simulink model "assignment_9"  (R2020b)
settings: Solver=VariableStepAuto  StartTime=0.0  StopTime=0.2  RelTol=1e-3
settings Model: Creator=Sudhanshu  LastModifiedBy=Sudhanshu

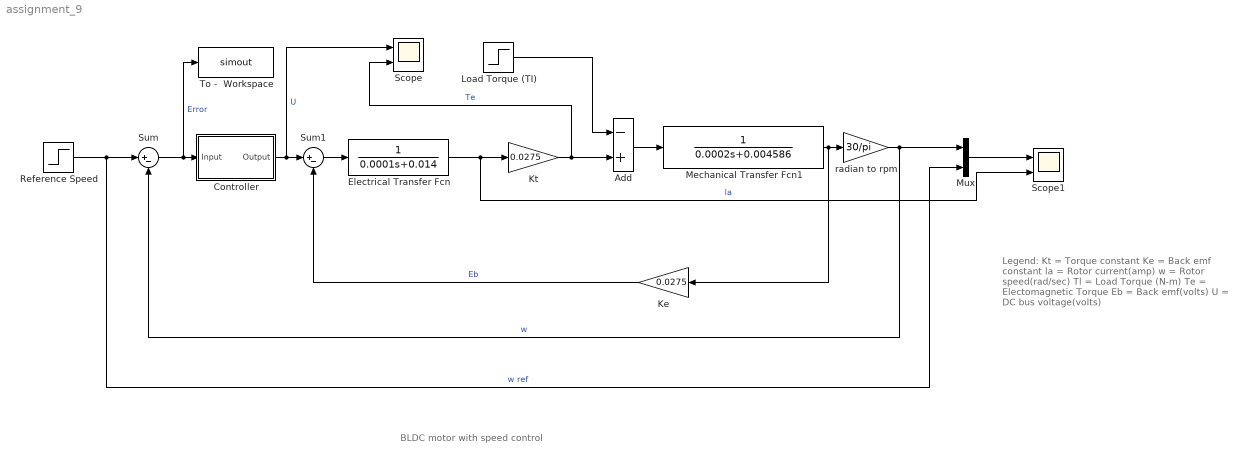
== system assignment_9 ==
  note: BLDC motor with speed control
  note: Legend:
      |
      | Kt = Torque constant
      | Ke = Back emf constant
      | la = Rotor current(amp)
      | w = Rotor speed(rad/sec)
      | Tl = Load Torque (N-m)
      | Te = Electomagnetic Torque
      | Eb = Back emf(volts)
      | U = DC bus voltage(volts)
  Add : Sum  Inputs=-+
  Controller : Subsystem
  Electrical Transfer Fcn : TransferFcn  Denominator=[0.0001 0.014]
  Ke : Gain  Gain=0.0275
  Kt : Gain  Gain=0.0275
  Load Torque (TI) : Step  Time=0.1  After=10  SampleTime=0  ZeroCross=off
  Mechanical Transfer Fcn1 : TransferFcn  Denominator=[0.0002 0.004586]
  Mux : Mux  Inputs=2
  Reference Speed : Step  Time=0  After=1500  SampleTime=0
  Scope : Scope  NumInputPorts=2
  Scope1 : Scope  NumInputPorts=2
  Sum : Sum  Inputs=|+-
  Sum1 : Sum  Inputs=|+-
  To -  Workspace : ToWorkspace  VariableName=simout  SaveFormat=Timeseries  SampleTime=-1
  radian to rpm : Gain  Gain=30/pi
  wires:
  Reference Speed/1 -> Mux/2, Sum/1  "w ref"
  Sum1/1 -> Electrical Transfer Fcn/1
  Sum/1 -> To -  Workspace/1, Controller/1(Input)  "Error"
  Controller/1(Output) -> Scope/1, Sum1/1  "U"
  Kt/1 -> Scope/2, Add/2  "Te"
  Load Torque (TI)/1 -> Add/1
  Add/1 -> Mechanical Transfer Fcn1/1
  Electrical Transfer Fcn/1 -> Scope1/2, Kt/1  "la"
  Ke/1 -> Sum1/2  "Eb"
  Mux/1 -> Scope1/1
  Mechanical Transfer Fcn1/1 -> Ke/1, radian to rpm/1
  radian to rpm/1 -> Mux/1, Sum/2  "w"

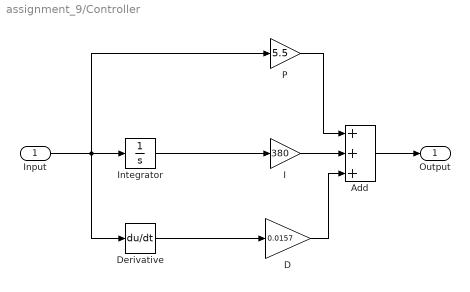
== system assignment_9/Controller ==
  Input : Inport
  Add : Sum  Inputs=+++
  D : Gain  Gain=0.0157
  Derivative : Derivative
  I : Gain  Gain=380
  Integrator : Integrator
  P : Gain  Gain=5.5
  Output : Outport
  wires:
  Input/1 -> Derivative/1, P/1, Integrator/1
  Add/1 -> Output/1
  I/1 -> Add/2
  P/1 -> Add/1
  D/1 -> Add/3
  Integrator/1 -> I/1
  Derivative/1 -> D/1
